simulink model "hw4_a"  (R2024b)
settings: Solver=FixedStepDiscrete  StartTime=0.0  StopTime=40  FixedStep=ts  RelTol=1e-3
values from neighbouring files (symbols this model uses):
  Am = in(5:7)    [diophantineSolver_custom.m]    (also in hw4_a.m = den)
  Ao = in(8:9)    [diophantineSolver_custom.m]    (also in hw4_a.m = [1 -0.15])
  den = den{1}    [hw4_a.m]
  noise_mean = 0    [hw4_a.m]
  noise_seed = round(rand*1e5)    [hw4_a.m]
  noise_variance = 0.5    [hw4_a.m]
  num = num(2:end)    [hw4_a.m]
  ts = 0.1    [hw4_a.m]
  X = [1 0.01]    [hw4_a.m]    (also in integralAction.m = in(9:10))
undefined symbols (not defined in the file or in its folder): dspblkCoreblockFVToolHelper, gcbh
settings Model: PauseTimes=25  PacingRate=0.900000  Creator=kemal  LastModifiedBy=kemal

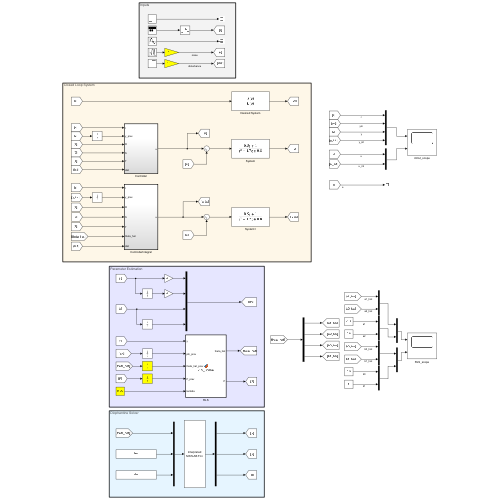
[thumbnail: Simulink's stored preview of the top-level diagram]
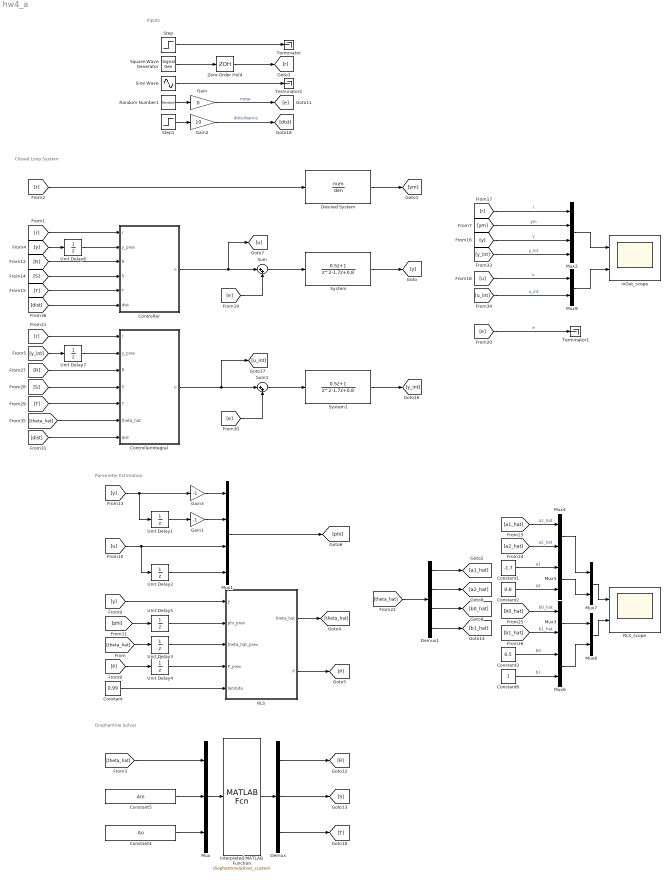
== system hw4_a ==
  note: Closed Loop System
  note: Parameter Estimation
  note: Inputs
  note: Diophantine Solver
  Constant : Constant  Value=0.99  SampleTime=ts
  Constant1 : Constant  Value=-1.7  SampleTime=ts
  Constant2 : Constant  Value=0.8  SampleTime=ts
  Constant3 : Constant  Value=0.5  SampleTime=ts
  Constant4 : Constant  Value=Ao  SampleTime=ts
  Constant5 : Constant  Value=Am  VectorParams1D=off  SampleTime=ts
  Constant6 : Constant  SampleTime=ts
  Controller : Subsystem  TreatAsAtomicUnit=on  SystemSampleTime=ts
  ControllerIntegral : Subsystem  TreatAsAtomicUnit=on  SystemSampleTime=ts
  Demux : Demux  Outputs=[2, 2, 2]
  Demux1 : Demux
  Desired System : DiscreteTransferFcn  LoadFcn=dspblkCoreblockFVToolHelper(gcbh,'load');  Numerator=num  Denominator=den
      settings: CopyFcn=dspblkCoreblockFVToolHelper(gcbh,'copy');  DeleteFcn=dspblkCoreblockFVToolHelper(gcbh,'close');  ModelCloseFcn=dspblkCoreblockFVToolHelper(gcbh,'close');  PreSaveFcn=dspblkCoreblockFVToolHelper(gcbh,'presave');  PostSaveFcn=dspblkCoreblockFVToolHelper(gcbh,'postsave');  CloseFcn=dspblkCoreblockFVToolHelper(gcbh,'close');
  Gain : Gain  Gain=0
  Gain1 : Gain  Gain=-1
  Gain2 : Gain  Gain=10
  Gain3 : Gain  Gain=-1
  Interpreted MATLAB Function : MATLABFcn  MATLABFcn=diophantineSolver_custom  OutputDimensions=6  Output1D=off
  Mux : Mux  Inputs=3
  Mux1 : Mux
  Mux2 : Mux
  Mux{3..9} (7 alike) : Mux  Inputs=2
  RLS : MATLAB Function  TreatAsAtomicUnit=on
  RLS_scope : Scope  NumInputPorts=2
  Random Number1 : RandomNumber  Mean=noise_mean  Variance=noise_variance  Seed=noise_seed  SampleTime=ts
  Sine Wave : Sin  Amplitude=25  Frequency=0.25  SampleTime=ts
  Square Wave Generator : SignalGenerator  WaveForm=square  Amplitude=-10  Frequency=1/20
  Step : Step  Time=0.1  After=5  SampleTime=ts
  Step1 : Step  Time=17  SampleTime=ts
  Sum : Sum  Inputs=|++
  Sum1 : Sum  Inputs=|++
  System : DiscreteTransferFcn  LoadFcn=dspblkCoreblockFVToolHelper(gcbh,'load');  Numerator=[0.5 1]  Denominator=[1 -1.7 0.8]
      settings: CopyFcn=dspblkCoreblockFVToolHelper(gcbh,'copy');  DeleteFcn=dspblkCoreblockFVToolHelper(gcbh,'close');  ModelCloseFcn=dspblkCoreblockFVToolHelper(gcbh,'close');  PreSaveFcn=dspblkCoreblockFVToolHelper(gcbh,'presave');  PostSaveFcn=dspblkCoreblockFVToolHelper(gcbh,'postsave');  CloseFcn=dspblkCoreblockFVToolHelper(gcbh,'close');
  System1 : DiscreteTransferFcn  LoadFcn=dspblkCoreblockFVToolHelper(gcbh,'load');  Numerator=[0.5 1]  Denominator=[1 -1.7 0.8]
      settings: CopyFcn=dspblkCoreblockFVToolHelper(gcbh,'copy');  DeleteFcn=dspblkCoreblockFVToolHelper(gcbh,'close');  ModelCloseFcn=dspblkCoreblockFVToolHelper(gcbh,'close');  PreSaveFcn=dspblkCoreblockFVToolHelper(gcbh,'presave');  PostSaveFcn=dspblkCoreblockFVToolHelper(gcbh,'postsave');  CloseFcn=dspblkCoreblockFVToolHelper(gcbh,'close');
  Terminator : Terminator
  Terminator1 : Terminator
  Terminator2 : Terminator
  Unit Delay{1..2,6..7} (4 alike) : UnitDelay  SampleTime=ts  HasFrameUpgradeWarning=on
  Unit Delay3 : UnitDelay  InitialCondition=[0.5 0.6 0.7 0.8]  SampleTime=ts  HasFrameUpgradeWarning=on
  Unit Delay4 : UnitDelay  InitialCondition=eye(4)*1000  SampleTime=ts  HasFrameUpgradeWarning=on
  Unit Delay5 : UnitDelay  InitialCondition=zeros(4,1)  SampleTime=ts  HasFrameUpgradeWarning=on
  Zero-Order Hold : ZeroOrderHold  SampleTime=ts
  inOut_scope : Scope  NumInputPorts=2
  wires:
  RLS/1(theta_hat) -> [theta_hat]
  [phi] -> Unit Delay5/1
  [theta_hat] -> Unit Delay3/1
  Mux1/1 -> [phi]
  RLS/2(P) -> [P]
  [y] -> Unit Delay1/1, Gain3/1
  Gain3/1 -> Mux1/1
  Constant/1 -> RLS/5(lambda)
  [y] -> RLS/1(y)
  [P] -> Unit Delay4/1
  Unit Delay4/1 -> RLS/4(P_prev)
  Unit Delay3/1 -> RLS/3(theta_hat_prev)
  Unit Delay5/1 -> RLS/2(phi_prev)
  System/1 -> [y]
  Desired System/1 -> [ym]
  Unit Delay1/1 -> Gain1/1
  Gain1/1 -> Mux1/2
  [u] -> Unit Delay2/1, Mux1/3
  Unit Delay2/1 -> Mux1/4
  Square Wave Generator/1 -> Zero-Order Hold/1
  Random Number1/1 -> Gain/1
  Demux/3 -> [T]
  Demux/2 -> [S]
  Demux/1 -> [R]
  Constant5/1 -> Mux/2
  Mux/1 -> Interpreted MATLAB Function/1
  Interpreted MATLAB Function/1 -> Demux/1
  [ym] -> Mux2/2  "ym"
  [y] -> Mux2/3  "y"
  [r] -> Mux2/1  "r"
  Mux2/1 -> inOut_scope/1
  Constant4/1 -> Mux/3
  Sum/1 -> System/1
  Gain/1 -> [e]  "noise"
  [r] -> Desired System/1
  [theta_hat] -> Mux/1
  [theta_hat] -> Demux1/1
  Demux1/1 -> [a1_hat]
  Demux1/2 -> [a2_hat]
  Demux1/3 -> [b0_hat]
  Demux1/4 -> [b1_hat]
  [a1_hat] -> Mux4/1  "a1_hat"
  [a2_hat] -> Mux4/2  "a2_hat"
  [b0_hat] -> Mux3/1  "b0_hat"
  [b1_hat] -> Mux3/2  "b1_hat"
  Constant2/1 -> Mux5/2  "a2"
  Constant3/1 -> Mux6/1  "b0"
  Constant6/1 -> Mux6/2  "b1"
  Constant1/1 -> Mux5/1  "a1"
  Mux7/1 -> RLS_scope/1
  Mux4/1 -> Mux7/1
  Mux5/1 -> Mux7/2
  Mux3/1 -> Mux8/1
  Mux6/1 -> Mux8/2
  Mux8/1 -> RLS_scope/2
  [e] -> Terminator1/1  "e"
  Step/1 -> Terminator/1
  Sine Wave/1 -> Terminator2/1
  Sum1/1 -> System1/1
  [e] -> Sum1/2
  [y_int] -> Mux2/4  "y_int"
  [u] -> Mux9/1  "u"
  [u_int] -> Mux9/2  "u_int"
  Mux9/1 -> inOut_scope/2
  [theta_hat] -> ControllerIntegral/6(theta_hat)
  [T] -> ControllerIntegral/5(T)
  [S] -> ControllerIntegral/4(S)
  [R] -> ControllerIntegral/3(R)
  [r] -> ControllerIntegral/1(r)
  Unit Delay7/1 -> ControllerIntegral/2(y_prev)
  [y_int] -> Unit Delay7/1
  ControllerIntegral/1(u) -> [u_int], Sum1/1
  [y] -> Unit Delay6/1
  [r] -> Controller/1(r)
  Unit Delay6/1 -> Controller/2(y_prev)
  [R] -> Controller/3(R)
  [S] -> Controller/4(S)
  [T] -> Controller/5(T)
  Controller/1(u) -> [u], Sum/1
  System1/1 -> [y_int]
  [dist] -> ControllerIntegral/7(dist)
  Step1/1 -> Gain2/1
  [dist] -> Controller/6(dist)
  Zero-Order Hold/1 -> [r]
  [e] -> Sum/2
  Gain2/1 -> [dist]  "disturbance"

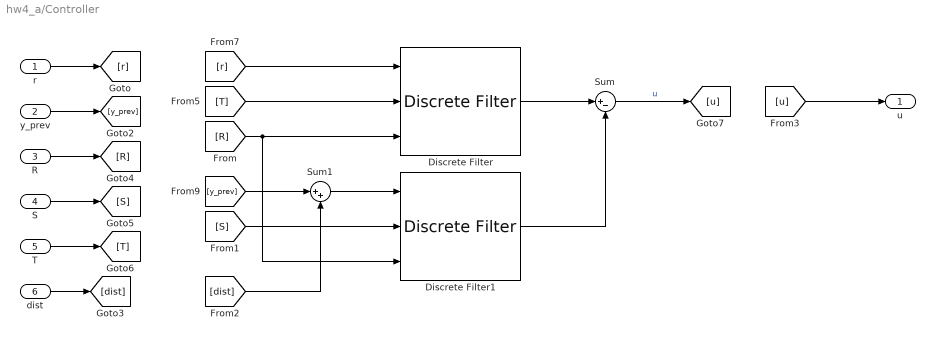
== system hw4_a/Controller ==
  r : Inport
  y_prev : Inport  Port=2
  R : Inport  Port=3
  S : Inport  Port=4
  T : Inport  Port=5
  dist : Inport  Port=6
  Discrete Filter : DiscreteFilter  LoadFcn=dspblkCoreblockFVToolHelper(gcbh,'load');  NumeratorSource=Input port  DenominatorSource=Input port  a0EqualsOne=on
      settings: CopyFcn=dspblkCoreblockFVToolHelper(gcbh,'copy');  DeleteFcn=dspblkCoreblockFVToolHelper(gcbh,'close');  ModelCloseFcn=dspblkCoreblockFVToolHelper(gcbh,'close');  PreSaveFcn=dspblkCoreblockFVToolHelper(gcbh,'presave');  PostSaveFcn=dspblkCoreblockFVToolHelper(gcbh,'postsave');  CloseFcn=dspblkCoreblockFVToolHelper(gcbh,'close');  InputPortMap=u0,p1,p3
  Discrete Filter1 : DiscreteFilter  LoadFcn=dspblkCoreblockFVToolHelper(gcbh,'load');  NumeratorSource=Input port  DenominatorSource=Input port  a0EqualsOne=on
      settings: CopyFcn=dspblkCoreblockFVToolHelper(gcbh,'copy');  DeleteFcn=dspblkCoreblockFVToolHelper(gcbh,'close');  ModelCloseFcn=dspblkCoreblockFVToolHelper(gcbh,'close');  PreSaveFcn=dspblkCoreblockFVToolHelper(gcbh,'presave');  PostSaveFcn=dspblkCoreblockFVToolHelper(gcbh,'postsave');  CloseFcn=dspblkCoreblockFVToolHelper(gcbh,'close');  InputPortMap=u0,p1,p3
  Sum : Sum  Inputs=|+-
  Sum1 : Sum  Inputs=|++
  u : Outport
  wires:
  Sum/1 -> [u]  "u"
  Discrete Filter1/1 -> Sum/2
  Discrete Filter/1 -> Sum/1
  [S] -> Discrete Filter1/2
  [r] -> Discrete Filter/1
  [R] -> Discrete Filter/3, Discrete Filter1/3
  [T] -> Discrete Filter/2
  [u] -> u/1
  T/1 -> [T]
  S/1 -> [S]
  R/1 -> [R]
  y_prev/1 -> [y_prev]
  r/1 -> [r]
  dist/1 -> [dist]
  Sum1/1 -> Discrete Filter1/1
  [y_prev] -> Sum1/1
  [dist] -> Sum1/2

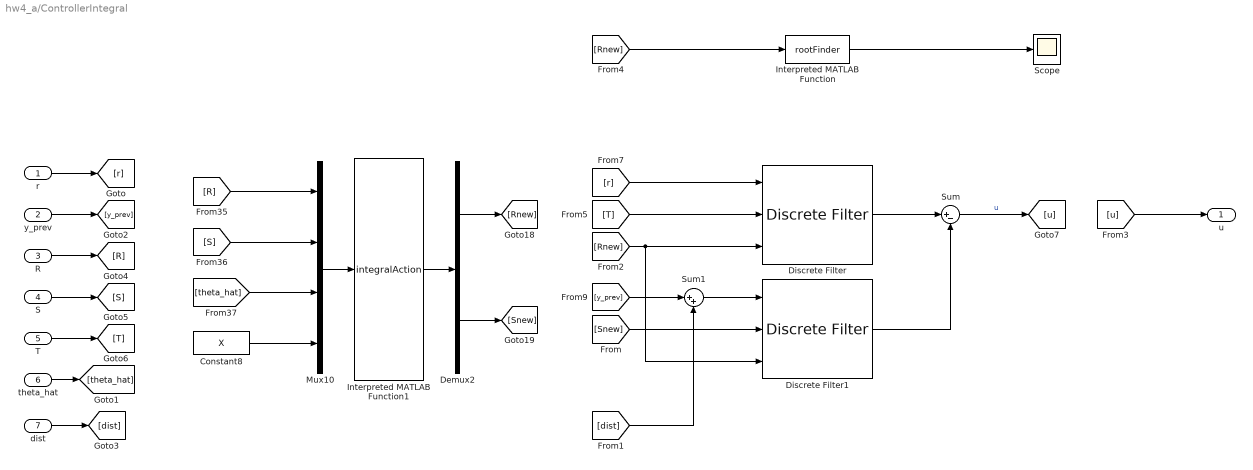
== system hw4_a/ControllerIntegral ==
  r : Inport
  y_prev : Inport  Port=2
  R : Inport  Port=3
  S : Inport  Port=4
  T : Inport  Port=5
  theta_hat : Inport  Port=6
  dist : Inport  Port=7
  Constant8 : Constant  Value=X  SampleTime=ts
  Demux2 : Demux  Outputs=[3, 3]
  Discrete Filter : DiscreteFilter  LoadFcn=dspblkCoreblockFVToolHelper(gcbh,'load');  NumeratorSource=Input port  DenominatorSource=Input port  a0EqualsOne=on
      settings: CopyFcn=dspblkCoreblockFVToolHelper(gcbh,'copy');  DeleteFcn=dspblkCoreblockFVToolHelper(gcbh,'close');  ModelCloseFcn=dspblkCoreblockFVToolHelper(gcbh,'close');  PreSaveFcn=dspblkCoreblockFVToolHelper(gcbh,'presave');  PostSaveFcn=dspblkCoreblockFVToolHelper(gcbh,'postsave');  CloseFcn=dspblkCoreblockFVToolHelper(gcbh,'close');  InputPortMap=u0,p1,p3
  Discrete Filter1 : DiscreteFilter  LoadFcn=dspblkCoreblockFVToolHelper(gcbh,'load');  NumeratorSource=Input port  DenominatorSource=Input port  a0EqualsOne=on
      settings: CopyFcn=dspblkCoreblockFVToolHelper(gcbh,'copy');  DeleteFcn=dspblkCoreblockFVToolHelper(gcbh,'close');  ModelCloseFcn=dspblkCoreblockFVToolHelper(gcbh,'close');  PreSaveFcn=dspblkCoreblockFVToolHelper(gcbh,'presave');  PostSaveFcn=dspblkCoreblockFVToolHelper(gcbh,'postsave');  CloseFcn=dspblkCoreblockFVToolHelper(gcbh,'close');  InputPortMap=u0,p1,p3
  Interpreted MATLAB Function : MATLABFcn  MATLABFcn=rootFinder  OutputDimensions=2  Output1D=off
  Interpreted MATLAB Function1 : MATLABFcn  MATLABFcn=integralAction  OutputDimensions=6  Output1D=off
  Mux10 : Mux
  Scope : Scope
  Sum : Sum  Inputs=|+-
  Sum1 : Sum  Inputs=|++
  u : Outport
  wires:
  Interpreted MATLAB Function/1 -> Scope/1
  [Rnew] -> Interpreted MATLAB Function/1
  dist/1 -> [dist]
  [dist] -> Sum1/2
  Sum1/1 -> Discrete Filter1/1
  r/1 -> [r]
  y_prev/1 -> [y_prev]
  R/1 -> [R]
  S/1 -> [S]
  T/1 -> [T]
  [u] -> u/1
  [T] -> Discrete Filter/2
  [Rnew] -> Discrete Filter1/3, Discrete Filter/3
  [r] -> Discrete Filter/1
  [Snew] -> Discrete Filter1/2
  [y_prev] -> Sum1/1
  Discrete Filter/1 -> Sum/1
  Discrete Filter1/1 -> Sum/2
  Sum/1 -> [u]  "u"
  theta_hat/1 -> [theta_hat]
  [R] -> Mux10/1
  [S] -> Mux10/2
  Constant8/1 -> Mux10/4
  [theta_hat] -> Mux10/3
  Mux10/1 -> Interpreted MATLAB Function1/1
  Demux2/2 -> [Snew]
  Interpreted MATLAB Function1/1 -> Demux2/1
  Demux2/1 -> [Rnew]

== matlab function hw4_a/RLS ==
  data: y input; theta_hat output; phi_prev input; theta_hat_prev input; P_prev input; lambda input; P output
function [theta_hat, P] = RLS_update(y, phi_prev, theta_hat_prev, P_prev, lambda)
    % Compute innovation
    epsilon = y - phi_prev' * theta_hat_prev;
     
    % Update covariance matrix
    P = (1/lambda) * (P_prev - (P_prev * (phi_prev * phi_prev') * P_prev) / ...
        (lambda + phi_prev' * P_prev * phi_prev));

    % Update parameter estimate
    theta_hat = theta_hat_prev + P * phi_prev * epsilon;
end
